simulink model "EStopLatch"  (R2026a)
settings: Solver=FixedStepDiscrete  StopTime=10  FixedStep=0.01
model workspace (MAT data in the model file):
  P.safety_io_poll_period = 0.1
  P.driver_states_update_frequency = 20
  P.safety_latch_reset_pulse = 0.1
  P.modbus_response_timeout = 0.15
  P.dt = 0.01
  P.link_delay = 0
  P.latch_reset_requires_zero = 0
  P.publish_phase = 0
Description:
  | As-built E-stop chain (rover_hardware_interface + safety PLC). Generated by scripts/build_estop_latch.m.
settings Model: Creator=potlo  LastModifiedBy=potlo
settings DataIOCC: LoadExternalInput=on

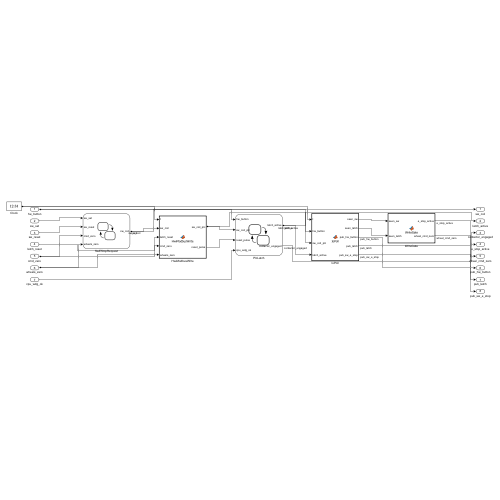
[thumbnail: Simulink's stored preview of the top-level diagram]
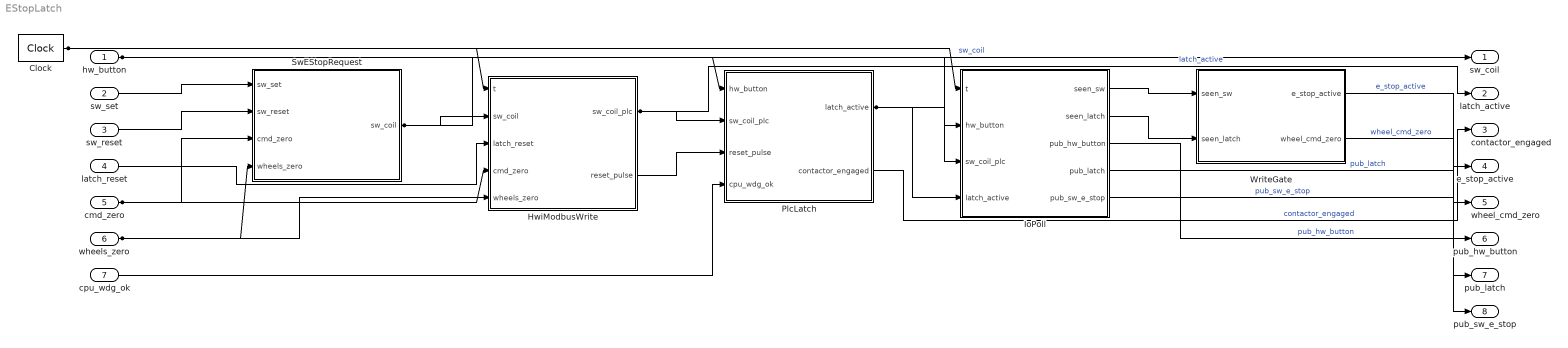
== system EStopLatch ==
  hw_button : Inport  Interpolate=off
  sw_set : Inport  Port=2  Interpolate=off
  sw_reset : Inport  Port=3  Interpolate=off
  latch_reset : Inport  Port=4  Interpolate=off
  cmd_zero : Inport  Port=5  Interpolate=off
  wheels_zero : Inport  Port=6  Interpolate=off
  cpu_wdg_ok : Inport  Port=7  Interpolate=off
  Clock : DigitalClock  SampleTime=0.01
  HwiModbusWrite : MATLAB Function  TreatAsAtomicUnit=on
  IoPoll : MATLAB Function  TreatAsAtomicUnit=on
  PlcLatch : Stateflow chart  TreatAsAtomicUnit=on
  SwEStopRequest : Stateflow chart  TreatAsAtomicUnit=on
  WriteGate : MATLAB Function  TreatAsAtomicUnit=on
  sw_coil : Outport
  latch_active : Outport  Port=2
  contactor_engaged : Outport  Port=3
  e_stop_active : Outport  Port=4
  wheel_cmd_zero : Outport  Port=5
  pub_hw_button : Outport  Port=6
  pub_latch : Outport  Port=7
  pub_sw_e_stop : Outport  Port=8
  wires:
  sw_set/1 -> SwEStopRequest/1(sw_set)
  sw_reset/1 -> SwEStopRequest/2(sw_reset)
  cmd_zero/1 -> SwEStopRequest/3(cmd_zero), HwiModbusWrite/4(cmd_zero)
  wheels_zero/1 -> SwEStopRequest/4(wheels_zero), HwiModbusWrite/5(wheels_zero)
  Clock/1 -> HwiModbusWrite/1(t), IoPoll/1(t)
  SwEStopRequest/1(sw_coil) -> HwiModbusWrite/2(sw_coil), sw_coil/1  "sw_coil"
  latch_reset/1 -> HwiModbusWrite/3(latch_reset)
  hw_button/1 -> PlcLatch/1(hw_button), IoPoll/2(hw_button)
  HwiModbusWrite/1(sw_coil_plc) -> PlcLatch/2(sw_coil_plc), IoPoll/3(sw_coil_plc)
  HwiModbusWrite/2(reset_pulse) -> PlcLatch/3(reset_pulse)
  cpu_wdg_ok/1 -> PlcLatch/4(cpu_wdg_ok)
  PlcLatch/1(latch_active) -> IoPoll/4(latch_active), latch_active/1  "latch_active"
  IoPoll/1(seen_sw) -> WriteGate/1(seen_sw)
  IoPoll/2(seen_latch) -> WriteGate/2(seen_latch)
  PlcLatch/2(contactor_engaged) -> contactor_engaged/1  "contactor_engaged"
  WriteGate/1(e_stop_active) -> e_stop_active/1  "e_stop_active"
  WriteGate/2(wheel_cmd_zero) -> wheel_cmd_zero/1  "wheel_cmd_zero"
  IoPoll/3(pub_hw_button) -> pub_hw_button/1  "pub_hw_button"
  IoPoll/4(pub_latch) -> pub_latch/1  "pub_latch"
  IoPoll/5(pub_sw_e_stop) -> pub_sw_e_stop/1  "pub_sw_e_stop"

== stateflow chart EStopLatch/PlcLatch ==
  settings: updateMethod=DISCRETE  sampleTime=0.01
  state Latched
    entry: latch_active = 1; contactor_engaged = 0;
  state Clear
    entry: latch_active = 0; contactor_engaged = 1;
  (default) -> Latched
  Latched -> Clear : [reset_pulse > 0.5 && ~(hw_button > 0.5 || sw_coil_plc > 0.5 || cpu_wdg_ok < 0.5)]
  Clear -> Latched : [(hw_button > 0.5 || sw_coil_plc > 0.5 || cpu_wdg_ok < 0.5)]
  data: hw_button input double; sw_coil_plc input double; reset_pulse input double; cpu_wdg_ok input double; latch_active output double; contactor_engaged output double

== matlab function EStopLatch/HwiModbusWrite ==
  data: t input; sw_coil_plc output; sw_coil input; latch_reset input; cmd_zero input; wheels_zero input; reset_pulse output; P parameter
function [sw_coil_plc, reset_pulse] = HwiModbusWrite(t, sw_coil, latch_reset, cmd_zero, wheels_zero, P)
persistent buf idx prev_req pulse_until
n = max(1, round(P.link_delay / P.dt) + 1);
if isempty(buf), buf = zeros(1, 64); idx = 1; prev_req = 0; pulse_until = -inf; end
buf(idx) = sw_coil;
sw_coil_plc = buf(mod(idx - n, 64) + 1);
idx = mod(idx, 64) + 1;
accept = P.latch_reset_requires_zero < 0.5 || (cmd_zero > 0.5 && wheels_zero > 0.5);
if latch_reset > 0.5 && prev_req < 0.5 && accept
    pulse_until = t + P.link_delay + P.safety_latch_reset_pulse;
end
prev_req = latch_reset;
reset_pulse = double(t >= pulse_until - P.safety_latch_reset_pulse - 1e-9 && t < pulse_until - 1e-9);

== stateflow chart EStopLatch/SwEStopRequest ==
  settings: updateMethod=DISCRETE  sampleTime=0.01
  state Released
    entry: sw_coil = 0;
  state Asserted
    entry: sw_coil = 1;
  (default) -> Released
  Released -> Asserted : [sw_set > 0.5]
  Asserted -> Released : [sw_reset > 0.5 && cmd_zero > 0.5 && wheels_zero > 0.5]
  data: sw_set input double; sw_reset input double; cmd_zero input double; wheels_zero input double; sw_coil output double

== matlab function EStopLatch/IoPoll ==
  data: t input; seen_sw output; hw_button input; sw_coil_plc input; latch_active input; seen_latch output; pub_hw_button output; pub_latch output; pub_sw_e_stop output; P parameter
function [seen_sw, seen_latch, pub_hw_button, pub_latch, pub_sw_e_stop] = IoPoll(t, hw_button, sw_coil_plc, latch_active, P)
persistent s_sw s_latch s_hw next_poll next_pub p_hw p_latch p_sw
if isempty(s_sw), s_sw = 0; s_latch = 1; s_hw = 0; next_poll = 0; next_pub = P.publish_phase; p_hw = 0; p_latch = 1; p_sw = 0; end
if t >= next_poll - 1e-9
    s_sw = sw_coil_plc; s_latch = latch_active; s_hw = hw_button;
    next_poll = t + P.safety_io_poll_period;
end
if t >= next_pub - 1e-9
    p_hw = s_hw; p_latch = s_latch; p_sw = s_sw;
    next_pub = t + 1 / P.driver_states_update_frequency;
end
seen_sw = s_sw; seen_latch = s_latch;
pub_hw_button = p_hw; pub_latch = p_latch; pub_sw_e_stop = p_sw;

== matlab function EStopLatch/WriteGate ==
  data: seen_sw input; e_stop_active output; seen_latch input; wheel_cmd_zero output
function [e_stop_active, wheel_cmd_zero] = WriteGate(seen_sw, seen_latch)
% RoverControlLoopUseCase::updateEStopActiveState / decideWriteCommand
e_stop_active = double(seen_sw > 0.5 || seen_latch > 0.5);
wheel_cmd_zero = e_stop_active;
